simulink model "ABS_model"  (R2024a)
settings: Solver=ode3  StartTime=0.0  StopTime=4.5  FixedStep=0.01  RelTol=1e-3
values from neighbouring files (symbols this model uses):
  ABS_mode = ABS_off    (= 0)    [test4_simulink.m]
  ABS_off = 0    [test4_simulink.m]
  C = 2.45    [test4_simulink.m]
  g = 9.81    [test4_simulink.m]
  I = 5    [test4_simulink.m]
  m = 1200    [test4_simulink.m]
  PBmax = 15    [test4_simulink.m]
  Re = 0.01    [test4_simulink.m]
  Rw = 0.001*(17*25.4+215*0.55*2)/2    (= 0.33415)    [test4_simulink.m]
  torque_scaling = 2000    [test4_simulink.m]
  v0 = 20    [test4_simulink.m]
libraries: simulink x1
settings Model: Creator=Corey  LastModifiedBy=Corey

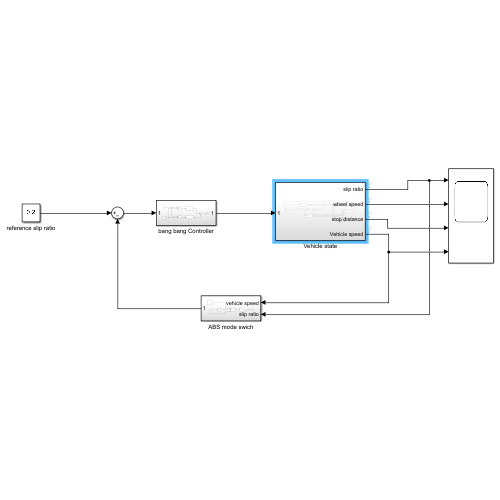
[thumbnail: Simulink's stored preview of the top-level diagram]
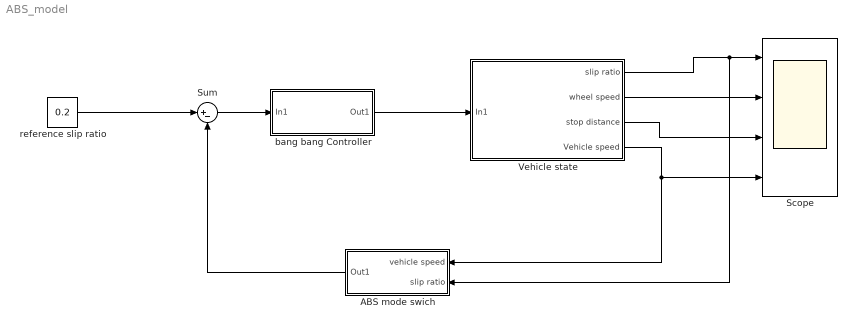
== system ABS_model ==
  ABS mode swich : Subsystem
  Scope : Scope  NumInputPorts=4
  Sum : Sum  Inputs=|+-
  Vehicle state : Subsystem
  bang bang Controller : Subsystem
  reference slip ratio : Constant  Value=0.2
  wires:
  reference slip ratio/1 -> Sum/1
  Sum/1 -> bang bang Controller/1(In1)
  bang bang Controller/1(Out1) -> Vehicle state/1(In1)
  ABS mode swich/1(Out1) -> Sum/2
  Vehicle state/1(slip ratio) -> ABS mode swich/2(slip ratio), Scope/1
  Vehicle state/2(wheel speed) -> Scope/2
  Vehicle state/3(stop distance) -> Scope/3
  Vehicle state/4(Vehicle speed) -> ABS mode swich/1(vehicle speed), Scope/4

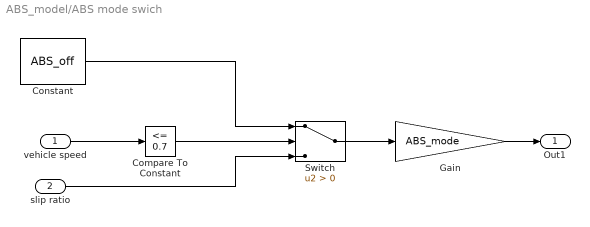
== system ABS_model/ABS mode swich ==
  vehicle speed : Inport
  slip ratio : Inport  Port=2
  Compare To Constant : simulink/Logic and Bit Operations/Compare To Constant  relop=<=  const=0.7  OutDataTypeStr=boolean
  Constant : Constant  Value=ABS_off
  Gain : Gain  Gain=ABS_mode
  Switch : Switch  Criteria=u2 > Threshold  SaturateOnIntegerOverflow=off  InputSameDT=off
  Out1 : Outport
  wires:
  Constant/1 -> Switch/1
  slip ratio/1 -> Switch/3
  Gain/1 -> Out1/1
  Switch/1 -> Gain/1
  vehicle speed/1 -> Compare To Constant/1
  Compare To Constant/1 -> Switch/2

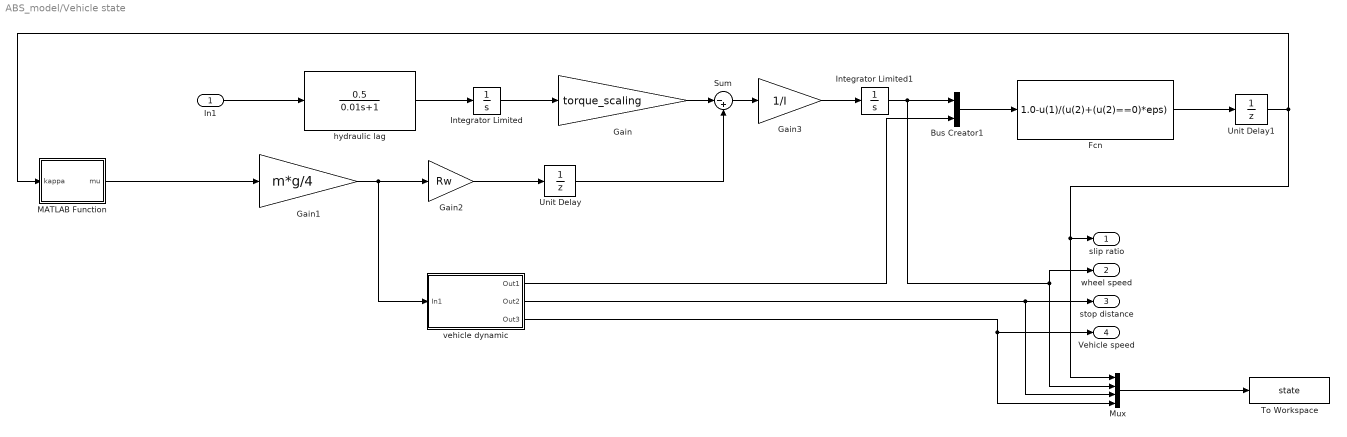
== system ABS_model/Vehicle state ==
  In1 : Inport
  Bus Creator1 : BusCreator  Inputs=2
  Fcn : Fcn  Expr=1.0-u(1)/(u(2)+(u(2)==0)*eps)
  Gain : Gain  Gain=torque_scaling
  Gain1 : Gain  Gain=m*g/4
  Gain2 : Gain  Gain=Rw
  Gain3 : Gain  Gain=1/I
  Integrator Limited : Integrator  LimitOutput=on  UpperSaturationLimit=PBmax  LowerSaturationLimit=0
  Integrator Limited1 : Integrator  InitialCondition=v0/Rw  LimitOutput=on  UpperSaturationLimit=200  LowerSaturationLimit=0  ZeroCross=off
  MATLAB Function : MATLAB Function  TreatAsAtomicUnit=on
  Mux : Mux
  Sum : Sum  Inputs=|-+
  To Workspace : ToWorkspace  VariableName=state  SaveFormat=Timeseries  SampleTime=-1
  Unit Delay : UnitDelay  SampleTime=-1  HasFrameUpgradeWarning=on
  Unit Delay1 : UnitDelay  SampleTime=-1  HasFrameUpgradeWarning=on
  hydraulic lag : TransferFcn  Numerator=[0.5]  Denominator=[0.01 1]
  vehicle dynamic : Subsystem
  slip ratio : Outport
  wheel speed : Outport  Port=2
  stop distance : Outport  Port=3
  Vehicle speed : Outport  Port=4
  wires:
  In1/1 -> hydraulic lag/1
  hydraulic lag/1 -> Integrator Limited/1
  Integrator Limited/1 -> Gain/1
  Gain/1 -> Sum/1
  Gain1/1 -> Gain2/1, vehicle dynamic/1(In1)
  Gain2/1 -> Unit Delay/1
  Unit Delay/1 -> Sum/2
  Sum/1 -> Gain3/1
  vehicle dynamic/1(Out1) -> Bus Creator1/2
  Fcn/1 -> Unit Delay1/1
  Unit Delay1/1 -> Mux/1, slip ratio/1, MATLAB Function/1(kappa)
  Integrator Limited1/1 -> Mux/2, wheel speed/1, Bus Creator1/1
  Gain3/1 -> Integrator Limited1/1
  vehicle dynamic/2(Out2) -> Mux/3, stop distance/1
  vehicle dynamic/3(Out3) -> Mux/4, Vehicle speed/1
  MATLAB Function/1(mu) -> Gain1/1
  Mux/1 -> To Workspace/1
  Bus Creator1/1 -> Fcn/1

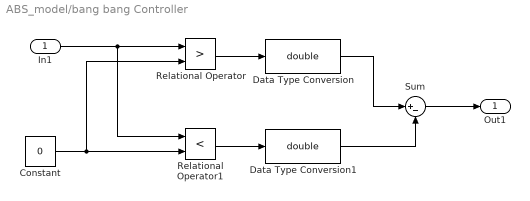
== system ABS_model/bang bang Controller ==
  In1 : Inport
  Constant : Constant  Value=0
  Data Type Conversion : DataTypeConversion  OutDataTypeStr=double  SaturateOnIntegerOverflow=off  RndMeth=Floor
  Data Type Conversion1 : DataTypeConversion  OutDataTypeStr=double  SaturateOnIntegerOverflow=off  RndMeth=Floor
  Relational Operator : RelationalOperator  Operator=>  OutDataTypeStr=boolean  RndMeth=Simplest  InputSameDT=off
  Relational Operator1 : RelationalOperator  Operator=<  OutDataTypeStr=boolean  RndMeth=Simplest  InputSameDT=off
  Sum : Sum  Inputs=|+-
  Out1 : Outport
  wires:
  Relational Operator/1 -> Data Type Conversion/1
  Relational Operator1/1 -> Data Type Conversion1/1
  Data Type Conversion/1 -> Sum/1
  Data Type Conversion1/1 -> Sum/2
  Sum/1 -> Out1/1
  In1/1 -> Relational Operator1/1, Relational Operator/1
  Constant/1 -> Relational Operator1/2, Relational Operator/2

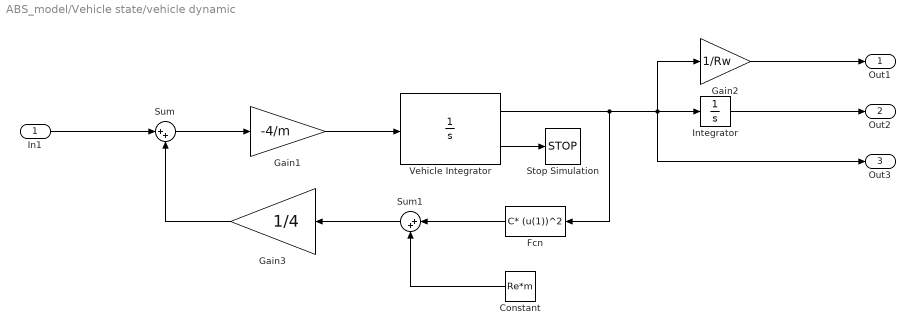
== system ABS_model/Vehicle state/vehicle dynamic ==
  In1 : Inport
  Constant : Constant  Value=Re*m
  Fcn : Fcn  Expr=C* (u(1))^2
  Gain1 : Gain  Gain=-4/m
  Gain2 : Gain  Gain=1/Rw
  Gain3 : Gain  Gain=1/4
  Integrator : Integrator
  Stop Simulation : Stop
  Sum : Sum  Inputs=|++
  Sum1 : Sum  Inputs=|++
  Vehicle Integrator : Integrator  InitialCondition=v0  LimitOutput=on  UpperSaturationLimit=500  LowerSaturationLimit=-1  ShowSaturationPort=on
  Out1 : Outport
  Out2 : Outport  Port=2
  Out3 : Outport  Port=3
  wires:
  Constant/1 -> Sum1/2
  Gain1/1 -> Vehicle Integrator/1
  Vehicle Integrator/1 -> Fcn/1, Out3/1, Gain2/1, Integrator/1
  Integrator/1 -> Out2/1
  Sum1/1 -> Gain3/1
  Gain3/1 -> Sum/2
  Fcn/1 -> Sum1/1
  Gain2/1 -> Out1/1
  Sum/1 -> Gain1/1
  In1/1 -> Sum/1
  Vehicle Integrator/2 -> Stop Simulation/1

== matlab function ABS_model/Vehicle state/MATLAB Function ==
  data: kappa input; mu output
function mu = magic_mu(kappa)
% Magic Formula tire model

% 參數（你給的）
D = 0.7;
C = 2.45;
B = 4;
E = 0.95;

% 保護 slip ratio 範圍，避免爆炸
kappa = max(min(kappa, 1), -1);

% Magic Formula 計算 μ
mu = D * sin( C * atan( B * kappa - E * (B * kappa - atan(B * kappa)) ) );
